simulink subsystem "FCS_Parameters"  (R2024b)
settings: Solver=VariableStepAuto  StartTime=0.0  StopTime=10.0  RelTol=1e-3
undefined symbols (not defined in the file): SimPar
settings Model: Creator=bmsimmon  LastModifiedBy=macheson
settings RTWCC: GPUComputeCapability=3.5

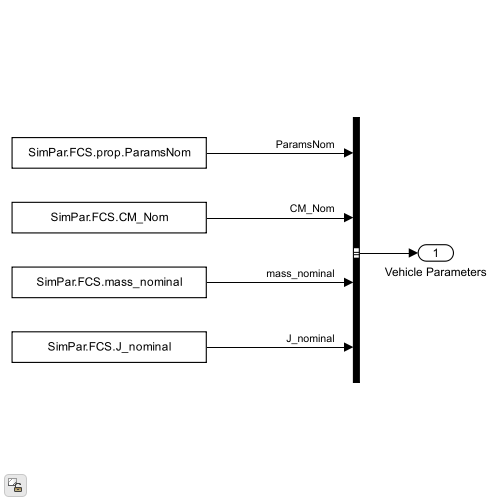
[thumbnail: Simulink's stored preview of the top-level diagram]
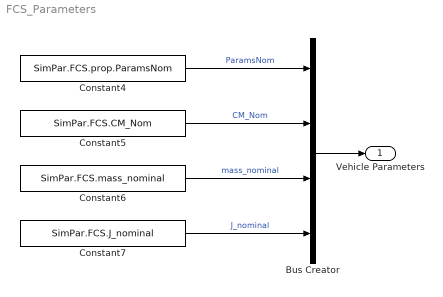
== system FCS_Parameters ==
  Bus Creator : BusCreator  Inputs=4
  Constant4 : Constant  Value=SimPar.FCS.prop.ParamsNom
  Constant5 : Constant  Value=SimPar.FCS.CM_Nom
  Constant6 : Constant  Value=SimPar.FCS.mass_nominal
  Constant7 : Constant  Value=SimPar.FCS.J_nominal
  Vehicle Parameters : Outport  VectorParamsAs1DForOutWhenUnconnected=off
  wires:
  Bus Creator/1 -> Vehicle Parameters/1
  Constant4/1 -> Bus Creator/1  "ParamsNom"
  Constant5/1 -> Bus Creator/2  "CM_Nom"
  Constant6/1 -> Bus Creator/3  "mass_nominal"
  Constant7/1 -> Bus Creator/4  "J_nominal"
